simulink model "asbhl20"  (R2016b)
settings: Solver=ode3  StartTime=0.0  StopTime=61  FixedStep=1/120  RelTol=1e-3  AbsTol=1e-6
PreLoadFcn:
  | load asbhl20data.mat
InitFcn:
  | timeSince1970.Value = etime(datevec(now),[1970, 1, 1, 0, 0, 0]);
values from neighbouring files (symbols this model uses):
  maxPackets = 100    [asbhl20data.mat]
  Tc = 0.0166666666667    [asbhl20GlobalChildrenData.mat]
  x_cg = 4.78635044684    [asbhl20data.mat]
undefined symbols (not defined in the file or in its folder): m, message, Receive, s, Send, sigbuilder_block
libraries: aerolibfltsims x5, simulink x4, asbhl20GPS x2, aerolibnav x2, asbhl20env x1, asbhl20airdata x1, asbhl20ralt x1, asbhl20commsys x1, asbhl20FADEC x1, asbhl20sensors x1, asbhl20LGC x1, asbhl20vehicle x1
(part 3 of 3)

== system asbhl20/HL-20 Vehicle Systems Model/Avionics/Left Avionics Bay/CPU C/Event Logging/Event Logging Wing ==
  In1 : Inport
  Bus Selector1 : BusSelector  OutputSignals=signal1,signal2,signal3,signal4,signal5.WR1_log,signal5.WR2_log,signal5.WL1_log,signal5.WL2_log
  Log WL1 Actuator Position Sensors : Subsystem  TreatAsAtomicUnit=on
  Log WL2 Actuator Position Sensors : Subsystem  TreatAsAtomicUnit=on
  Log WR1 Actuator Position Sensors : Subsystem  TreatAsAtomicUnit=on
  Log WR2 Actuator Position Sensors : Subsystem  TreatAsAtomicUnit=on
  wires:
  [WR1_log] -> Log WR1 Actuator Position Sensors/Enable
  In1/1 -> Bus Selector1/1
  [WR2_log] -> Log WR2 Actuator Position Sensors/Enable
  [WL1_log] -> Log WL1 Actuator Position Sensors/Enable
  [WL2_log] -> Log WL2 Actuator Position Sensors/Enable
  Bus Selector1/1 -> Log WR1 Actuator Position Sensors/1(In1)  "<signal1>"
  Bus Selector1/2 -> Log WR2 Actuator Position Sensors/1(In1)  "<signal2>"
  Bus Selector1/3 -> Log WL1 Actuator Position Sensors/1(In1)  "<signal3>"
  Bus Selector1/4 -> Log WL2 Actuator Position Sensors/1(In1)  "<signal4>"
  Bus Selector1/5 -> [WR1_log]  "<WR1_log>"
  Bus Selector1/6 -> [WR2_log]  "<WR2_log>"
  Bus Selector1/7 -> [WL1_log]  "<WL1_log>"
  Bus Selector1/8 -> [WL2_log]  "<WL2_log>"

== system asbhl20/HL-20 Vehicle Systems Model/Avionics/Left Avionics Bay/CPU C/Event Logging/Event Logging Wing Hydraulic ==
  In1 : Inport
  Bus Selector : BusSelector  OutputSignals=signal1,signal2,signal3,signal4.H1_log,signal4.H2_log,signal4.H3_log
  Log Hydraulic System 1 Sensors : Subsystem  TreatAsAtomicUnit=on
  Log Hydraulic System 2 Sensors : Subsystem  TreatAsAtomicUnit=on
  Log Hydraulic System 3 Sensors : Subsystem  TreatAsAtomicUnit=on
  wires:
  [H1_log] -> Log Hydraulic System 1 Sensors/Enable
  In1/1 -> Bus Selector/1
  [H2_log] -> Log Hydraulic System 2 Sensors/Enable
  [H3_log] -> Log Hydraulic System 3 Sensors/Enable
  Bus Selector/1 -> Log Hydraulic System 1 Sensors/1(In1)  "<signal1>"
  Bus Selector/2 -> Log Hydraulic System 2 Sensors/1(In1)  "<signal2>"
  Bus Selector/3 -> Log Hydraulic System 3 Sensors/1(In1)  "<signal3>"
  Bus Selector/4 -> [H1_log]  "<H1_log>"
  Bus Selector/5 -> [H2_log]  "<H2_log>"
  Bus Selector/6 -> [H3_log]  "<H3_log>"

== system asbhl20/HL-20 Vehicle Systems Model/Avionics/Right Avionics Bay/CPU A/Event Logging/Event Logging Left ==
  In1 : Inport
  Bus Selector : BusSelector  OutputSignals=signal1,signal2,signal3,signal4,signal5.LU1_log,signal5.LU2_log,signal5.LL1_log,signal5.LL2_log
  Log LL1 Actuator Position Sensors : Subsystem  TreatAsAtomicUnit=on
  Log LL2 Actuator Position Sensors : Subsystem  TreatAsAtomicUnit=on
  Log LU1 Actuator Position Sensors : Subsystem  TreatAsAtomicUnit=on
  Log LU2 Actuator Position Sensors : Subsystem  TreatAsAtomicUnit=on
  wires:
  [LU1_log] -> Log LU1 Actuator Position Sensors/Enable
  In1/1 -> Bus Selector/1
  [LU2_log] -> Log LU2 Actuator Position Sensors/Enable
  [LL1_log] -> Log LL1 Actuator Position Sensors/Enable
  [LL2_log] -> Log LL2 Actuator Position Sensors/Enable
  Bus Selector/1 -> Log LU1 Actuator Position Sensors/1(In1)  "<signal1>"
  Bus Selector/2 -> Log LU2 Actuator Position Sensors/1(In1)  "<signal2>"
  Bus Selector/3 -> Log LL1 Actuator Position Sensors/1(In1)  "<signal3>"
  Bus Selector/4 -> Log LL2 Actuator Position Sensors/1(In1)  "<signal4>"
  Bus Selector/5 -> [LU1_log]  "<LU1_log>"
  Bus Selector/6 -> [LU2_log]  "<LU2_log>"
  Bus Selector/7 -> [LL1_log]  "<LL1_log>"
  Bus Selector/8 -> [LL2_log]  "<LL2_log>"

== system asbhl20/HL-20 Vehicle Systems Model/Avionics/Right Avionics Bay/CPU A/Event Logging/Event Logging Lower Hydraulic ==
  In1 : Inport
  Bus Selector : BusSelector  OutputSignals=signal1,signal2,signal3,signal4.H7_log,signal4.H8_log,signal4.H9_log
  Log Hydraulic System 1 Sensors : Subsystem  TreatAsAtomicUnit=on
  Log Hydraulic System 2 Sensors : Subsystem  TreatAsAtomicUnit=on
  Log Hydraulic System 3 Sensors : Subsystem  TreatAsAtomicUnit=on
  wires:
  [H7_log] -> Log Hydraulic System 1 Sensors/Enable
  In1/1 -> Bus Selector/1
  [H8_log] -> Log Hydraulic System 2 Sensors/Enable
  [H9_log] -> Log Hydraulic System 3 Sensors/Enable
  Bus Selector/1 -> Log Hydraulic System 1 Sensors/1(In1)  "<signal1>"
  Bus Selector/2 -> Log Hydraulic System 2 Sensors/1(In1)  "<signal2>"
  Bus Selector/3 -> Log Hydraulic System 3 Sensors/1(In1)  "<signal3>"
  Bus Selector/4 -> [H7_log]  "<H7_log>"
  Bus Selector/5 -> [H8_log]  "<H8_log>"
  Bus Selector/6 -> [H9_log]  "<H9_log>"

== system asbhl20/HL-20 Vehicle Systems Model/Avionics/Right Avionics Bay/CPU A/Event Logging/Event Logging Right ==
  In1 : Inport
  Bus Selector : BusSelector  OutputSignals=signal1,signal2,signal3,signal4,signal5.RU1_log,signal5.RU2_log,signal5.RL1_log,signal5.RL2_log
  Log RL1 Actuator Position Sensors : Subsystem  TreatAsAtomicUnit=on
  Log RL2 Actuator Position Sensors : Subsystem  TreatAsAtomicUnit=on
  Log RU1 Actuator Position Sensors : Subsystem  TreatAsAtomicUnit=on
  Log RU2 Actuator Position Sensors : Subsystem  TreatAsAtomicUnit=on
  wires:
  Bus Selector/4 -> Log RL2 Actuator Position Sensors/1(In1)  "<signal4>"
  Bus Selector/3 -> Log RL1 Actuator Position Sensors/1(In1)  "<signal3>"
  Bus Selector/2 -> Log RU2 Actuator Position Sensors/1(In1)  "<signal2>"
  Bus Selector/1 -> Log RU1 Actuator Position Sensors/1(In1)  "<signal1>"
  [RL2_log] -> Log RL2 Actuator Position Sensors/Enable
  [RL1_log] -> Log RL1 Actuator Position Sensors/Enable
  [RU2_log] -> Log RU2 Actuator Position Sensors/Enable
  In1/1 -> Bus Selector/1
  [RU1_log] -> Log RU1 Actuator Position Sensors/Enable
  Bus Selector/5 -> [RU1_log]  "<RU1_log>"
  Bus Selector/6 -> [RU2_log]  "<RU2_log>"
  Bus Selector/7 -> [RL1_log]  "<RL1_log>"
  Bus Selector/8 -> [RL2_log]  "<RL2_log>"

== system asbhl20/HL-20 Vehicle Systems Model/Avionics/Right Avionics Bay/CPU A/Event Logging/Event Logging Upper Hydraulic ==
  In1 : Inport
  Bus Selector : BusSelector  OutputSignals=signal1,signal2,signal3,signal4.H4_log,signal4.H5_log,signal4.H6_log
  Log Hydraulic System 1 Sensors : Subsystem  TreatAsAtomicUnit=on
  Log Hydraulic System 2 Sensors : Subsystem  TreatAsAtomicUnit=on
  Log Hydraulic System 3 Sensors : Subsystem  TreatAsAtomicUnit=on
  wires:
  Bus Selector/3 -> Log Hydraulic System 3 Sensors/1(In1)  "<signal3>"
  Bus Selector/2 -> Log Hydraulic System 2 Sensors/1(In1)  "<signal2>"
  Bus Selector/1 -> Log Hydraulic System 1 Sensors/1(In1)  "<signal1>"
  [H6_log] -> Log Hydraulic System 3 Sensors/Enable
  [H5_log] -> Log Hydraulic System 2 Sensors/Enable
  In1/1 -> Bus Selector/1
  [H4_log] -> Log Hydraulic System 1 Sensors/Enable
  Bus Selector/4 -> [H4_log]  "<H4_log>"
  Bus Selector/5 -> [H5_log]  "<H5_log>"
  Bus Selector/6 -> [H6_log]  "<H6_log>"

== system asbhl20/HL-20 Vehicle Systems Model/Avionics/Right Avionics Bay/CPU A/Event Logging/Event Logging Wing ==
  In1 : Inport
  Bus Selector1 : BusSelector  OutputSignals=signal1,signal2,signal3,signal4,signal5.WR1_log,signal5.WR2_log,signal5.WL1_log,signal5.WL2_log
  Log WL1 Actuator Position Sensors : Subsystem  TreatAsAtomicUnit=on
  Log WL2 Actuator Position Sensors : Subsystem  TreatAsAtomicUnit=on
  Log WR1 Actuator Position Sensors : Subsystem  TreatAsAtomicUnit=on
  Log WR2 Actuator Position Sensors : Subsystem  TreatAsAtomicUnit=on
  wires:
  [WR1_log] -> Log WR1 Actuator Position Sensors/Enable
  In1/1 -> Bus Selector1/1
  [WR2_log] -> Log WR2 Actuator Position Sensors/Enable
  [WL1_log] -> Log WL1 Actuator Position Sensors/Enable
  [WL2_log] -> Log WL2 Actuator Position Sensors/Enable
  Bus Selector1/1 -> Log WR1 Actuator Position Sensors/1(In1)  "<signal1>"
  Bus Selector1/2 -> Log WR2 Actuator Position Sensors/1(In1)  "<signal2>"
  Bus Selector1/3 -> Log WL1 Actuator Position Sensors/1(In1)  "<signal3>"
  Bus Selector1/4 -> Log WL2 Actuator Position Sensors/1(In1)  "<signal4>"
  Bus Selector1/5 -> [WR1_log]  "<WR1_log>"
  Bus Selector1/6 -> [WR2_log]  "<WR2_log>"
  Bus Selector1/7 -> [WL1_log]  "<WL1_log>"
  Bus Selector1/8 -> [WL2_log]  "<WL2_log>"

== system asbhl20/HL-20 Vehicle Systems Model/Avionics/Right Avionics Bay/CPU A/Event Logging/Event Logging Wing Hydraulic ==
  In1 : Inport
  Bus Selector : BusSelector  OutputSignals=signal1,signal2,signal3,signal4.H1_log,signal4.H2_log,signal4.H3_log
  Log Hydraulic System 1 Sensors : Subsystem  TreatAsAtomicUnit=on
  Log Hydraulic System 2 Sensors : Subsystem  TreatAsAtomicUnit=on
  Log Hydraulic System 3 Sensors : Subsystem  TreatAsAtomicUnit=on
  wires:
  [H1_log] -> Log Hydraulic System 1 Sensors/Enable
  In1/1 -> Bus Selector/1
  [H2_log] -> Log Hydraulic System 2 Sensors/Enable
  [H3_log] -> Log Hydraulic System 3 Sensors/Enable
  Bus Selector/1 -> Log Hydraulic System 1 Sensors/1(In1)  "<signal1>"
  Bus Selector/2 -> Log Hydraulic System 2 Sensors/1(In1)  "<signal2>"
  Bus Selector/3 -> Log Hydraulic System 3 Sensors/1(In1)  "<signal3>"
  Bus Selector/4 -> [H1_log]  "<H1_log>"
  Bus Selector/5 -> [H2_log]  "<H2_log>"
  Bus Selector/6 -> [H3_log]  "<H3_log>"

== system asbhl20/HL-20 Vehicle Systems Model/Avionics/Left Avionics Bay/CPU B/Event Logging/Event Logging Left/Log LL1 Actuator Position Sensors ==
  In1 : Inport
  Enable : EnablePort
  To Workspace : ToWorkspace  VariableName=LL1log_CPU_B  SaveFormat=Structure With Time  SampleTime=-1
  wires:
  In1/1 -> To Workspace/1  "R_log"

== system asbhl20/HL-20 Vehicle Systems Model/Avionics/Left Avionics Bay/CPU B/Event Logging/Event Logging Left/Log LL2 Actuator Position Sensors ==
  In1 : Inport
  Enable : EnablePort
  To Workspace : ToWorkspace  VariableName=LL2_log_CPU_B  SaveFormat=Structure With Time  SampleTime=-1
  wires:
  In1/1 -> To Workspace/1  "LL2_log"

== system asbhl20/HL-20 Vehicle Systems Model/Avionics/Left Avionics Bay/CPU B/Event Logging/Event Logging Left/Log LU1 Actuator Position Sensors ==
  In1 : Inport
  Enable : EnablePort
  To Workspace : ToWorkspace  VariableName=LU1_log_CPU_B  SaveFormat=Structure With Time  SampleTime=-1
  wires:
  In1/1 -> To Workspace/1  "LU1_log"

== system asbhl20/HL-20 Vehicle Systems Model/Avionics/Left Avionics Bay/CPU B/Event Logging/Event Logging Left/Log LU2 Actuator Position Sensors ==
  In1 : Inport
  Enable : EnablePort
  To Workspace : ToWorkspace  VariableName=LU2_log_CPU_B  SaveFormat=Structure With Time  SampleTime=-1
  wires:
  In1/1 -> To Workspace/1  "LU2_log"

== system asbhl20/HL-20 Vehicle Systems Model/Avionics/Left Avionics Bay/CPU B/Event Logging/Event Logging Lower Hydraulic/Log Hydraulic System 1 Sensors ==
  In1 : Inport
  Enable : EnablePort
  To Workspace : ToWorkspace  VariableName=H7_log_CPU_B  SaveFormat=Structure With Time  SampleTime=-1
  wires:
  In1/1 -> To Workspace/1

== system asbhl20/HL-20 Vehicle Systems Model/Avionics/Left Avionics Bay/CPU B/Event Logging/Event Logging Lower Hydraulic/Log Hydraulic System 2 Sensors ==
  In1 : Inport
  Enable : EnablePort
  To Workspace : ToWorkspace  VariableName=H8_log_CPU_B  SaveFormat=Structure With Time  SampleTime=-1
  wires:
  In1/1 -> To Workspace/1  "H8_log"

== system asbhl20/HL-20 Vehicle Systems Model/Avionics/Left Avionics Bay/CPU B/Event Logging/Event Logging Lower Hydraulic/Log Hydraulic System 3 Sensors ==
  In1 : Inport
  Enable : EnablePort
  To Workspace : ToWorkspace  VariableName=H9_log_CPU_B  SaveFormat=Structure With Time  SampleTime=-1
  wires:
  In1/1 -> To Workspace/1  "H9_log"

== system asbhl20/HL-20 Vehicle Systems Model/Avionics/Left Avionics Bay/CPU B/Event Logging/Event Logging Right/Log RL1 Actuator Position Sensors ==
  In1 : Inport
  Enable : EnablePort
  To Workspace : ToWorkspace  VariableName=RL1log_CPU_B  SaveFormat=Structure With Time  SampleTime=-1
  wires:
  In1/1 -> To Workspace/1  "RL1_log"

== system asbhl20/HL-20 Vehicle Systems Model/Avionics/Left Avionics Bay/CPU B/Event Logging/Event Logging Right/Log RL2 Actuator Position Sensors ==
  In1 : Inport
  Enable : EnablePort
  To Workspace : ToWorkspace  VariableName=RL2_log_CPU_B  SaveFormat=Structure With Time  SampleTime=-1
  wires:
  In1/1 -> To Workspace/1  "RL2_log"

== system asbhl20/HL-20 Vehicle Systems Model/Avionics/Left Avionics Bay/CPU B/Event Logging/Event Logging Right/Log RU1 Actuator Position Sensors ==
  In1 : Inport
  Enable : EnablePort
  To Workspace : ToWorkspace  VariableName=RU1_log_CPU_B  SaveFormat=Structure With Time  SampleTime=-1
  wires:
  In1/1 -> To Workspace/1  "RU1_log"

== system asbhl20/HL-20 Vehicle Systems Model/Avionics/Left Avionics Bay/CPU B/Event Logging/Event Logging Right/Log RU2 Actuator Position Sensors ==
  In1 : Inport
  Enable : EnablePort
  To Workspace : ToWorkspace  VariableName=RU2_log_CPU_B  SaveFormat=Structure With Time  SampleTime=-1
  wires:
  In1/1 -> To Workspace/1  "RU2_log"

== system asbhl20/HL-20 Vehicle Systems Model/Avionics/Left Avionics Bay/CPU B/Event Logging/Event Logging Upper Hydraulic/Log Hydraulic System 1 Sensors ==
  In1 : Inport
  Enable : EnablePort
  To Workspace : ToWorkspace  VariableName=H4_log_CPU_B  SaveFormat=Structure With Time  SampleTime=-1
  wires:
  In1/1 -> To Workspace/1

== system asbhl20/HL-20 Vehicle Systems Model/Avionics/Left Avionics Bay/CPU B/Event Logging/Event Logging Upper Hydraulic/Log Hydraulic System 2 Sensors ==
  In1 : Inport
  Enable : EnablePort
  To Workspace : ToWorkspace  VariableName=H5_log_CPU_B  SaveFormat=Structure With Time  SampleTime=-1
  wires:
  In1/1 -> To Workspace/1  "H5_log"

== system asbhl20/HL-20 Vehicle Systems Model/Avionics/Left Avionics Bay/CPU B/Event Logging/Event Logging Upper Hydraulic/Log Hydraulic System 3 Sensors ==
  In1 : Inport
  Enable : EnablePort
  To Workspace : ToWorkspace  VariableName=H6_log_CPU_B  SaveFormat=Structure With Time  SampleTime=-1
  wires:
  In1/1 -> To Workspace/1  "H6_log"

== system asbhl20/HL-20 Vehicle Systems Model/Avionics/Left Avionics Bay/CPU B/Event Logging/Event Logging Wing/Log WL1 Actuator Position Sensors ==
  In1 : Inport
  Enable : EnablePort
  To Workspace : ToWorkspace  VariableName=WL1log_CPU_B  SaveFormat=Structure With Time  SampleTime=-1
  wires:
  In1/1 -> To Workspace/1  "WL1_log"

== system asbhl20/HL-20 Vehicle Systems Model/Avionics/Left Avionics Bay/CPU B/Event Logging/Event Logging Wing/Log WL2 Actuator Position Sensors ==
  In1 : Inport
  Enable : EnablePort
  To Workspace : ToWorkspace  VariableName=WL2_log_CPU_B  SaveFormat=Structure With Time  SampleTime=-1
  wires:
  In1/1 -> To Workspace/1  "WL2_log"

== system asbhl20/HL-20 Vehicle Systems Model/Avionics/Left Avionics Bay/CPU B/Event Logging/Event Logging Wing/Log WR1 Actuator Position Sensors ==
  In1 : Inport
  Enable : EnablePort
  To Workspace : ToWorkspace  VariableName=WR1_log_CPU_B  SaveFormat=Structure With Time  SampleTime=-1
  wires:
  In1/1 -> To Workspace/1  "WR1_log"

== system asbhl20/HL-20 Vehicle Systems Model/Avionics/Left Avionics Bay/CPU B/Event Logging/Event Logging Wing/Log WR2 Actuator Position Sensors ==
  In1 : Inport
  Enable : EnablePort
  To Workspace : ToWorkspace  VariableName=WR2_log_CPU_B  SaveFormat=Structure With Time  SampleTime=-1
  wires:
  In1/1 -> To Workspace/1  "WR2_log"

== system asbhl20/HL-20 Vehicle Systems Model/Avionics/Left Avionics Bay/CPU B/Event Logging/Event Logging Wing Hydraulic/Log Hydraulic System 1 Sensors ==
  In1 : Inport
  Enable : EnablePort
  To Workspace : ToWorkspace  VariableName=H1_log_CPU_B  SaveFormat=Structure With Time  SampleTime=-1
  wires:
  In1/1 -> To Workspace/1

== system asbhl20/HL-20 Vehicle Systems Model/Avionics/Left Avionics Bay/CPU B/Event Logging/Event Logging Wing Hydraulic/Log Hydraulic System 2 Sensors ==
  In1 : Inport
  Enable : EnablePort
  To Workspace : ToWorkspace  VariableName=H2_log_CPU_B  SaveFormat=Structure With Time  SampleTime=-1
  wires:
  In1/1 -> To Workspace/1  "H2_log"

== system asbhl20/HL-20 Vehicle Systems Model/Avionics/Left Avionics Bay/CPU B/Event Logging/Event Logging Wing Hydraulic/Log Hydraulic System 3 Sensors ==
  In1 : Inport
  Enable : EnablePort
  To Workspace : ToWorkspace  VariableName=H3_log_CPU_B  SaveFormat=Structure With Time  SampleTime=-1
  wires:
  In1/1 -> To Workspace/1  "H3_log"

== system asbhl20/HL-20 Vehicle Systems Model/Avionics/Left Avionics Bay/CPU C/Event Logging/Event Logging Left/Log LL1 Actuator Position Sensors ==
  In1 : Inport
  Enable : EnablePort
  To Workspace : ToWorkspace  VariableName=LL1log_CPU_C  SaveFormat=Structure With Time  SampleTime=-1
  wires:
  In1/1 -> To Workspace/1  "R_log"

== system asbhl20/HL-20 Vehicle Systems Model/Avionics/Left Avionics Bay/CPU C/Event Logging/Event Logging Left/Log LL2 Actuator Position Sensors ==
  In1 : Inport
  Enable : EnablePort
  To Workspace : ToWorkspace  VariableName=LL2_log_CPU_C  SaveFormat=Structure With Time  SampleTime=-1
  wires:
  In1/1 -> To Workspace/1  "LL2_log"

== system asbhl20/HL-20 Vehicle Systems Model/Avionics/Left Avionics Bay/CPU C/Event Logging/Event Logging Left/Log LU1 Actuator Position Sensors ==
  In1 : Inport
  Enable : EnablePort
  To Workspace : ToWorkspace  VariableName=LU1_log_CPU_C  SaveFormat=Structure With Time  SampleTime=-1
  wires:
  In1/1 -> To Workspace/1  "LU1_log"

== system asbhl20/HL-20 Vehicle Systems Model/Avionics/Left Avionics Bay/CPU C/Event Logging/Event Logging Left/Log LU2 Actuator Position Sensors ==
  In1 : Inport
  Enable : EnablePort
  To Workspace : ToWorkspace  VariableName=LU2_log_CPU_C  SaveFormat=Structure With Time  SampleTime=-1
  wires:
  In1/1 -> To Workspace/1  "LU2_log"

== system asbhl20/HL-20 Vehicle Systems Model/Avionics/Left Avionics Bay/CPU C/Event Logging/Event Logging Lower Hydraulic/Log Hydraulic System 1 Sensors ==
  In1 : Inport
  Enable : EnablePort
  To Workspace : ToWorkspace  VariableName=H7_log_CPU_C  SaveFormat=Structure With Time  SampleTime=-1
  wires:
  In1/1 -> To Workspace/1

== system asbhl20/HL-20 Vehicle Systems Model/Avionics/Left Avionics Bay/CPU C/Event Logging/Event Logging Lower Hydraulic/Log Hydraulic System 2 Sensors ==
  In1 : Inport
  Enable : EnablePort
  To Workspace : ToWorkspace  VariableName=H8_log_CPU_C  SaveFormat=Structure With Time  SampleTime=-1
  wires:
  In1/1 -> To Workspace/1  "H8_log"

== system asbhl20/HL-20 Vehicle Systems Model/Avionics/Left Avionics Bay/CPU C/Event Logging/Event Logging Lower Hydraulic/Log Hydraulic System 3 Sensors ==
  In1 : Inport
  Enable : EnablePort
  To Workspace : ToWorkspace  VariableName=H9_log_CPU_C  SaveFormat=Structure With Time  SampleTime=-1
  wires:
  In1/1 -> To Workspace/1  "H9_log"

== system asbhl20/HL-20 Vehicle Systems Model/Avionics/Left Avionics Bay/CPU C/Event Logging/Event Logging Right/Log RL1 Actuator Position Sensors ==
  In1 : Inport
  Enable : EnablePort
  To Workspace : ToWorkspace  VariableName=RL1log_CPU_C  SaveFormat=Structure With Time  SampleTime=-1
  wires:
  In1/1 -> To Workspace/1  "RL1_log"

== system asbhl20/HL-20 Vehicle Systems Model/Avionics/Left Avionics Bay/CPU C/Event Logging/Event Logging Right/Log RL2 Actuator Position Sensors ==
  In1 : Inport
  Enable : EnablePort
  To Workspace : ToWorkspace  VariableName=RL2_log_CPU_C  SaveFormat=Structure With Time  SampleTime=-1
  wires:
  In1/1 -> To Workspace/1  "RL2_log"

== system asbhl20/HL-20 Vehicle Systems Model/Avionics/Left Avionics Bay/CPU C/Event Logging/Event Logging Right/Log RU1 Actuator Position Sensors ==
  In1 : Inport
  Enable : EnablePort
  To Workspace : ToWorkspace  VariableName=RU1_log_CPU_C  SaveFormat=Structure With Time  SampleTime=-1
  wires:
  In1/1 -> To Workspace/1  "RU1_log"

== system asbhl20/HL-20 Vehicle Systems Model/Avionics/Left Avionics Bay/CPU C/Event Logging/Event Logging Right/Log RU2 Actuator Position Sensors ==
  In1 : Inport
  Enable : EnablePort
  To Workspace : ToWorkspace  VariableName=RU2_log_CPU_C  SaveFormat=Structure With Time  SampleTime=-1
  wires:
  In1/1 -> To Workspace/1  "RU2_log"

== system asbhl20/HL-20 Vehicle Systems Model/Avionics/Left Avionics Bay/CPU C/Event Logging/Event Logging Upper Hydraulic/Log Hydraulic System 1 Sensors ==
  In1 : Inport
  Enable : EnablePort
  To Workspace : ToWorkspace  VariableName=H4_log_CPU_C  SaveFormat=Structure With Time  SampleTime=-1
  wires:
  In1/1 -> To Workspace/1

== system asbhl20/HL-20 Vehicle Systems Model/Avionics/Left Avionics Bay/CPU C/Event Logging/Event Logging Upper Hydraulic/Log Hydraulic System 2 Sensors ==
  In1 : Inport
  Enable : EnablePort
  To Workspace : ToWorkspace  VariableName=H5_log_CPU_C  SaveFormat=Structure With Time  SampleTime=-1
  wires:
  In1/1 -> To Workspace/1  "H5_log"

== system asbhl20/HL-20 Vehicle Systems Model/Avionics/Left Avionics Bay/CPU C/Event Logging/Event Logging Upper Hydraulic/Log Hydraulic System 3 Sensors ==
  In1 : Inport
  Enable : EnablePort
  To Workspace : ToWorkspace  VariableName=H6_log_CPU_C  SaveFormat=Structure With Time  SampleTime=-1
  wires:
  In1/1 -> To Workspace/1  "H6_log"

== system asbhl20/HL-20 Vehicle Systems Model/Avionics/Left Avionics Bay/CPU C/Event Logging/Event Logging Wing/Log WL1 Actuator Position Sensors ==
  In1 : Inport
  Enable : EnablePort
  To Workspace : ToWorkspace  VariableName=WL1log_CPU_C  SaveFormat=Structure With Time  SampleTime=-1
  wires:
  In1/1 -> To Workspace/1  "WL1_log"

== system asbhl20/HL-20 Vehicle Systems Model/Avionics/Left Avionics Bay/CPU C/Event Logging/Event Logging Wing/Log WL2 Actuator Position Sensors ==
  In1 : Inport
  Enable : EnablePort
  To Workspace : ToWorkspace  VariableName=WL2_log_CPU_C  SaveFormat=Structure With Time  SampleTime=-1
  wires:
  In1/1 -> To Workspace/1  "WL2_log"

== system asbhl20/HL-20 Vehicle Systems Model/Avionics/Left Avionics Bay/CPU C/Event Logging/Event Logging Wing/Log WR1 Actuator Position Sensors ==
  In1 : Inport
  Enable : EnablePort
  To Workspace : ToWorkspace  VariableName=WR1_log_CPU_C  SaveFormat=Structure With Time  SampleTime=-1
  wires:
  In1/1 -> To Workspace/1  "WR1_log"

== system asbhl20/HL-20 Vehicle Systems Model/Avionics/Left Avionics Bay/CPU C/Event Logging/Event Logging Wing/Log WR2 Actuator Position Sensors ==
  In1 : Inport
  Enable : EnablePort
  To Workspace : ToWorkspace  VariableName=WR2_log_CPU_C  SaveFormat=Structure With Time  SampleTime=-1
  wires:
  In1/1 -> To Workspace/1  "WR2_log"

== system asbhl20/HL-20 Vehicle Systems Model/Avionics/Left Avionics Bay/CPU C/Event Logging/Event Logging Wing Hydraulic/Log Hydraulic System 1 Sensors ==
  In1 : Inport
  Enable : EnablePort
  To Workspace : ToWorkspace  VariableName=H1_log_CPU_C  SaveFormat=Structure With Time  SampleTime=-1
  wires:
  In1/1 -> To Workspace/1

== system asbhl20/HL-20 Vehicle Systems Model/Avionics/Left Avionics Bay/CPU C/Event Logging/Event Logging Wing Hydraulic/Log Hydraulic System 2 Sensors ==
  In1 : Inport
  Enable : EnablePort
  To Workspace : ToWorkspace  VariableName=H2_log_CPU_C  SaveFormat=Structure With Time  SampleTime=-1
  wires:
  In1/1 -> To Workspace/1  "H2_log"

== system asbhl20/HL-20 Vehicle Systems Model/Avionics/Left Avionics Bay/CPU C/Event Logging/Event Logging Wing Hydraulic/Log Hydraulic System 3 Sensors ==
  In1 : Inport
  Enable : EnablePort
  To Workspace : ToWorkspace  VariableName=H3_log_CPU_C  SaveFormat=Structure With Time  SampleTime=-1
  wires:
  In1/1 -> To Workspace/1  "H3_log"

== system asbhl20/HL-20 Vehicle Systems Model/Avionics/Right Avionics Bay/CPU A/Event Logging/Event Logging Left/Log LL1 Actuator Position Sensors ==
  In1 : Inport
  Enable : EnablePort
  To Workspace : ToWorkspace  VariableName=LL1log_CPU_A  SaveFormat=Structure With Time  SampleTime=-1
  wires:
  In1/1 -> To Workspace/1  "R_log"

== system asbhl20/HL-20 Vehicle Systems Model/Avionics/Right Avionics Bay/CPU A/Event Logging/Event Logging Left/Log LL2 Actuator Position Sensors ==
  In1 : Inport
  Enable : EnablePort
  To Workspace : ToWorkspace  VariableName=LL2_log_CPU_A  SaveFormat=Structure With Time  SampleTime=-1
  wires:
  In1/1 -> To Workspace/1  "LL2_log"

== system asbhl20/HL-20 Vehicle Systems Model/Avionics/Right Avionics Bay/CPU A/Event Logging/Event Logging Left/Log LU1 Actuator Position Sensors ==
  In1 : Inport
  Enable : EnablePort
  To Workspace : ToWorkspace  VariableName=LU1_log_CPU_A  SaveFormat=Structure With Time  SampleTime=-1
  wires:
  In1/1 -> To Workspace/1  "LU1_log"

== system asbhl20/HL-20 Vehicle Systems Model/Avionics/Right Avionics Bay/CPU A/Event Logging/Event Logging Left/Log LU2 Actuator Position Sensors ==
  In1 : Inport
  Enable : EnablePort
  To Workspace : ToWorkspace  VariableName=LU2_log_CPU_A  SaveFormat=Structure With Time  SampleTime=-1
  wires:
  In1/1 -> To Workspace/1  "LU2_log"

== system asbhl20/HL-20 Vehicle Systems Model/Avionics/Right Avionics Bay/CPU A/Event Logging/Event Logging Lower Hydraulic/Log Hydraulic System 1 Sensors ==
  In1 : Inport
  Enable : EnablePort
  To Workspace : ToWorkspace  VariableName=H7_log_CPU_A  SaveFormat=Structure With Time  SampleTime=-1
  wires:
  In1/1 -> To Workspace/1

== system asbhl20/HL-20 Vehicle Systems Model/Avionics/Right Avionics Bay/CPU A/Event Logging/Event Logging Lower Hydraulic/Log Hydraulic System 2 Sensors ==
  In1 : Inport
  Enable : EnablePort
  To Workspace : ToWorkspace  VariableName=H8_log_CPU_A  SaveFormat=Structure With Time  SampleTime=-1
  wires:
  In1/1 -> To Workspace/1  "H8_log"

== system asbhl20/HL-20 Vehicle Systems Model/Avionics/Right Avionics Bay/CPU A/Event Logging/Event Logging Lower Hydraulic/Log Hydraulic System 3 Sensors ==
  In1 : Inport
  Enable : EnablePort
  To Workspace : ToWorkspace  VariableName=H9_log_CPU_A  SaveFormat=Structure With Time  SampleTime=-1
  wires:
  In1/1 -> To Workspace/1  "H9_log"

== system asbhl20/HL-20 Vehicle Systems Model/Avionics/Right Avionics Bay/CPU A/Event Logging/Event Logging Right/Log RL1 Actuator Position Sensors ==
  In1 : Inport
  Enable : EnablePort
  To Workspace : ToWorkspace  VariableName=RL1log_CPU_A  SaveFormat=Structure With Time  SampleTime=-1
  wires:
  In1/1 -> To Workspace/1  "RL1_log"

== system asbhl20/HL-20 Vehicle Systems Model/Avionics/Right Avionics Bay/CPU A/Event Logging/Event Logging Right/Log RL2 Actuator Position Sensors ==
  In1 : Inport
  Enable : EnablePort
  To Workspace : ToWorkspace  VariableName=RL2_log_CPU_A  SaveFormat=Structure With Time  SampleTime=-1
  wires:
  In1/1 -> To Workspace/1  "RL2_log"

== system asbhl20/HL-20 Vehicle Systems Model/Avionics/Right Avionics Bay/CPU A/Event Logging/Event Logging Right/Log RU1 Actuator Position Sensors ==
  In1 : Inport
  Enable : EnablePort
  To Workspace : ToWorkspace  VariableName=RU1_log_CPU_A  SaveFormat=Structure With Time  SampleTime=-1
  wires:
  In1/1 -> To Workspace/1  "RU1_log"

== system asbhl20/HL-20 Vehicle Systems Model/Avionics/Right Avionics Bay/CPU A/Event Logging/Event Logging Right/Log RU2 Actuator Position Sensors ==
  In1 : Inport
  Enable : EnablePort
  To Workspace : ToWorkspace  VariableName=RU2_log_CPU_A  SaveFormat=Structure With Time  SampleTime=-1
  wires:
  In1/1 -> To Workspace/1  "RU2_log"

== system asbhl20/HL-20 Vehicle Systems Model/Avionics/Right Avionics Bay/CPU A/Event Logging/Event Logging Upper Hydraulic/Log Hydraulic System 1 Sensors ==
  In1 : Inport
  Enable : EnablePort
  To Workspace : ToWorkspace  VariableName=H4_log_CPU_A  SaveFormat=Structure With Time  SampleTime=-1
  wires:
  In1/1 -> To Workspace/1

== system asbhl20/HL-20 Vehicle Systems Model/Avionics/Right Avionics Bay/CPU A/Event Logging/Event Logging Upper Hydraulic/Log Hydraulic System 2 Sensors ==
  In1 : Inport
  Enable : EnablePort
  To Workspace : ToWorkspace  VariableName=H5_log_CPU_A  SaveFormat=Structure With Time  SampleTime=-1
  wires:
  In1/1 -> To Workspace/1  "H5_log"

== system asbhl20/HL-20 Vehicle Systems Model/Avionics/Right Avionics Bay/CPU A/Event Logging/Event Logging Upper Hydraulic/Log Hydraulic System 3 Sensors ==
  In1 : Inport
  Enable : EnablePort
  To Workspace : ToWorkspace  VariableName=H6_log_CPU_A  SaveFormat=Structure With Time  SampleTime=-1
  wires:
  In1/1 -> To Workspace/1  "H6_log"

== system asbhl20/HL-20 Vehicle Systems Model/Avionics/Right Avionics Bay/CPU A/Event Logging/Event Logging Wing/Log WL1 Actuator Position Sensors ==
  In1 : Inport
  Enable : EnablePort
  To Workspace : ToWorkspace  VariableName=WL1log_CPU_A  SaveFormat=Structure With Time  SampleTime=-1
  wires:
  In1/1 -> To Workspace/1  "WL1_log"

== system asbhl20/HL-20 Vehicle Systems Model/Avionics/Right Avionics Bay/CPU A/Event Logging/Event Logging Wing/Log WL2 Actuator Position Sensors ==
  In1 : Inport
  Enable : EnablePort
  To Workspace : ToWorkspace  VariableName=WL2_log_CPU_A  SaveFormat=Structure With Time  SampleTime=-1
  wires:
  In1/1 -> To Workspace/1  "WL2_log"

== system asbhl20/HL-20 Vehicle Systems Model/Avionics/Right Avionics Bay/CPU A/Event Logging/Event Logging Wing/Log WR1 Actuator Position Sensors ==
  In1 : Inport
  Enable : EnablePort
  To Workspace : ToWorkspace  VariableName=WR1_log_CPU_A  SaveFormat=Structure With Time  SampleTime=-1
  wires:
  In1/1 -> To Workspace/1  "WR1_log"

== system asbhl20/HL-20 Vehicle Systems Model/Avionics/Right Avionics Bay/CPU A/Event Logging/Event Logging Wing/Log WR2 Actuator Position Sensors ==
  In1 : Inport
  Enable : EnablePort
  To Workspace : ToWorkspace  VariableName=WR2_log_CPU_A  SaveFormat=Structure With Time  SampleTime=-1
  wires:
  In1/1 -> To Workspace/1  "WR2_log"

== system asbhl20/HL-20 Vehicle Systems Model/Avionics/Right Avionics Bay/CPU A/Event Logging/Event Logging Wing Hydraulic/Log Hydraulic System 1 Sensors ==
  In1 : Inport
  Enable : EnablePort
  To Workspace : ToWorkspace  VariableName=H1_log_CPU_A  SaveFormat=Structure With Time  SampleTime=-1
  wires:
  In1/1 -> To Workspace/1

== system asbhl20/HL-20 Vehicle Systems Model/Avionics/Right Avionics Bay/CPU A/Event Logging/Event Logging Wing Hydraulic/Log Hydraulic System 2 Sensors ==
  In1 : Inport
  Enable : EnablePort
  To Workspace : ToWorkspace  VariableName=H2_log_CPU_A  SaveFormat=Structure With Time  SampleTime=-1
  wires:
  In1/1 -> To Workspace/1  "H2_log"

== system asbhl20/HL-20 Vehicle Systems Model/Avionics/Right Avionics Bay/CPU A/Event Logging/Event Logging Wing Hydraulic/Log Hydraulic System 3 Sensors ==
  In1 : Inport
  Enable : EnablePort
  To Workspace : ToWorkspace  VariableName=H3_log_CPU_A  SaveFormat=Structure With Time  SampleTime=-1
  wires:
  In1/1 -> To Workspace/1  "H3_log"
